simulink model "Aufgabe1"  (R2023a)
settings: Solver=VariableStepAuto  StartTime=0.0  StopTime=10.0  RelTol=1e-3
settings Model: Creator=splas  LastModifiedBy=splas
settings SolverCC: ShapePreserveControl=EnableAll

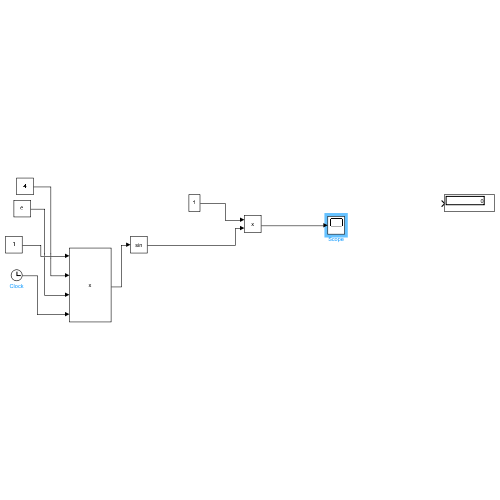
[thumbnail: Simulink's stored preview of the top-level diagram]
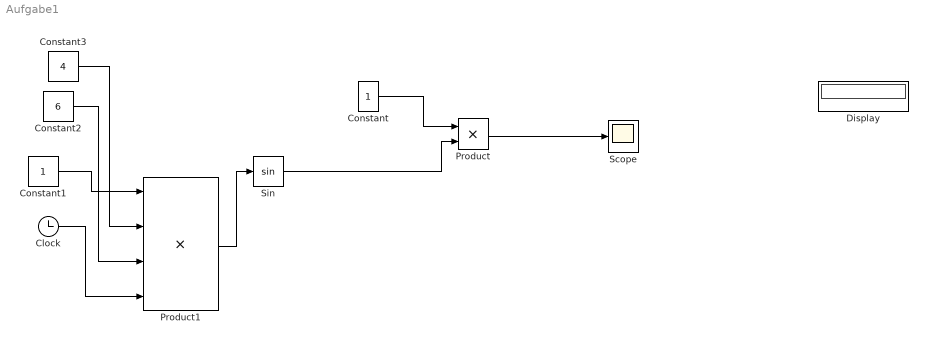
== system Aufgabe1 ==
  Clock : Clock
  Constant : Constant
  Constant1 : Constant
  Constant2 : Constant  Value=6
  Constant3 : Constant  Value=4
  Display : Display
  Product : Product
  Product1 : Product  Inputs=4
  Scope : Scope
  Sin : Trigonometry
  wires:
  Constant/1 -> Product/1
  Sin/1 -> Product/2
  Product1/1 -> Sin/1
  Clock/1 -> Product1/4
  Constant1/1 -> Product1/1
  Constant2/1 -> Product1/3
  Constant3/1 -> Product1/2
  Product/1 -> Scope/1
